simulink model "test_delfttyre_sti_cleat"  (Simulink 6.4)
settings: Solver=ode45  SolverMode=SingleTasking  StartTime=0.0  StopTime=0.5  FixedStep=0.00025  MaxStep=0.001  RelTol=1e-4  AbsTol=1e-4
values from neighbouring files (symbols this model uses):
  axle_z = typarr_struct.DIMENSION.UNLOADED_RADIUS - varinf(varinf_ptr.IDEFL)    [run_cleat_example_reduced_input_tpf.m]
  IYY_wheel = IYY-BELT_IYY+RIMROTIN+TRGROTIN    [run_cleat_example_reduced_input_tpf.m]
  Omega0 = Vx/varinf(varinf_ptr.IREF)    [run_cleat_example_reduced_input_tpf.m]
  Vx = 40/3.6    (= 11.1111111111)    [run_cleat_example_reduced_input_tpf.m]
libraries: simulink x4, Delft_Tyre_sm1glib x2, Delft_Tyre_dtlib x2
settings Model: Creator=schmeitzajc  LastModifiedBy=hofstadrhmtvd  ExtModeTrigMode=oneshot  ExtModeArmWhenConnect=off
settings SolverCC: InitialStep=0.001
settings DataIOCC: LimitDataPoints=off  SignalLoggingName=sigsOut
settings OptimizationCC: BooleanDataType=off
settings DebuggingCC: SolverPrmCheckMsg=none  StrictBusMsg=ErrorLevel1
settings HardwareCC: TargetHWDeviceType=32-bit Generic  TargetUnknown=on  ProdEqTarget=off

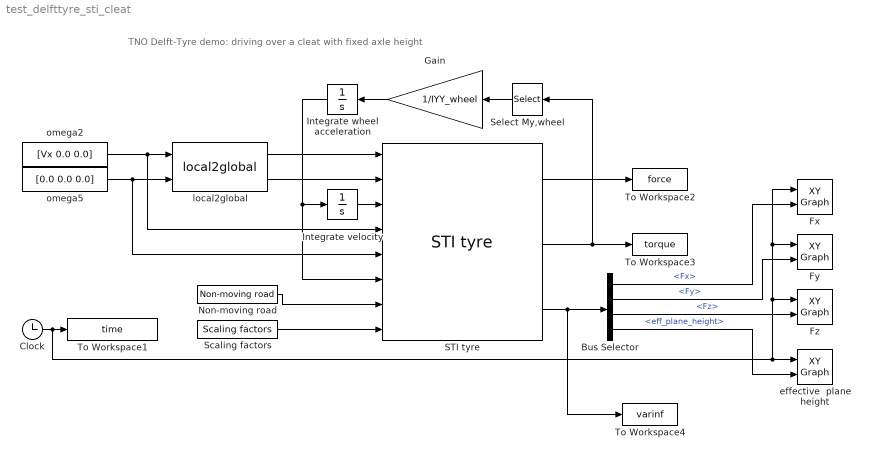
== system test_delfttyre_sti_cleat ==
  note: TNO Delft-Tyre demo: driving over a cleat with fixed axle height
  Bus Selector : BusSelector  OutputSignals=Fx,Fy,Fz,eff_plane_height
  Clock : Clock
      settings: Decimation=10
  Fx : simulink/Sinks/XY Graph  SystemSampleTime=-1  xmin=0  xmax=0.5  ymin=-2000  ymax=2000  st=-1
  Fy : simulink/Sinks/XY Graph  SystemSampleTime=-1  xmin=0  xmax=0.5  ymin=-1000  ymax=1000  st=-1
  Fz : simulink/Sinks/XY Graph  SystemSampleTime=-1  xmin=0  xmax=0.5  ymin=0  ymax=10000  st=-1
  Gain : Gain  Orientation=left  Gain=1/IYY_wheel  ParameterDataType=fixdt(1,16,0)  ParameterScaling=[]  OutDataType=fixdt(1,16,0)  OutScaling=[]
  Integrate velocity : Integrator
  Integrate wheel acceleration : Integrator  Orientation=left  InitialCondition=Omega0
  Non-moving road : Delft_Tyre_sm1glib/SimMechanics 1G/Non-moving road  Tag=Non-moving road  SystemSampleTime=-1  dummy=off
  STI tyre : Delft_Tyre_dtlib/Simulink/STI tyre  Tag=STI tyre  SystemSampleTime=-1  idtyre=1  tpfname=tpfname  rdfname=rdfname  side_mode=(3xxx) symmetric  cnt_mode=(x5xx) 3D short wavelength road contact  dyn_mode=(xx4x) rigid ring + initial statics  mf_mode=(xxx4) combined  use_mode=1e8  disp_debug=off
  Scaling factors : Delft_Tyre_sm1glib/SimMechanics 1G/Scaling factors  Tag=Scaling factors  SystemSampleTime=-1  LMUX=1  LKX=1  LMUY=1  LKY=1  LKYC=1  LTR=1  LKZC=1
  Select My,wheel : Selector  Orientation=left  Elements=2  Rows=2  InputPortWidth=3  OutputPortSize=[(-2)]
  To Workspace1 : ToWorkspace  VariableName=time  SampleTime=-1  SaveFormat=Array
  To Workspace2 : ToWorkspace  VariableName=force  SampleTime=-1  SaveFormat=Array
  To Workspace3 : ToWorkspace  VariableName=torque  SampleTime=-1  SaveFormat=Array
  To Workspace4 : ToWorkspace  VariableName=varinf  SampleTime=-1  SaveFormat=Array
  effective  plane height : simulink/Sinks/XY Graph  SystemSampleTime=-1  xmin=0  xmax=0.5  ymin=-0.05  ymax=0.05  st=-1
  local2global : Delft_Tyre_dtlib/Simulink/local2global  Tag=local2global  SystemSampleTime=-1  init_pos=[0 0 axle_z]  init_angle=[0 0 0]
  omega2 : Constant  Value=[Vx 0.0 0.0]  OutDataType=fixdt(1,16,0)  ConRadixGroup=Use specified scaling  OutScaling=[]  SampleTime=inf  FramePeriod=inf
  omega5 : Constant  Value=[0.0 0.0 0.0]  OutDataType=fixdt(1,16,0)  ConRadixGroup=Use specified scaling  OutScaling=[]  SampleTime=inf  FramePeriod=inf
  wires:
  STI tyre/1 -> To Workspace2/1
  Clock/1 -> To Workspace1/1, effective  plane height/1, Fz/1, Fx/1, Fy/1
  omega2/1 -> STI tyre/4, local2global/1
  Integrate wheel acceleration/1 -> Integrate velocity/1, STI tyre/6
  omega5/1 -> STI tyre/5, local2global/2
  STI tyre/2 -> To Workspace3/1, Select My,wheel/1
  STI tyre/3 -> Bus Selector/1, To Workspace4/1
  local2global/1 -> STI tyre/1
  local2global/2 -> STI tyre/2
  Integrate velocity/1 -> STI tyre/3
  Scaling factors/1 -> STI tyre/8
  Bus Selector/1 -> Fx/2  "<Fx>"
  Bus Selector/3 -> Fz/2  "<Fz>"
  Bus Selector/4 -> effective  plane height/2  "<eff_plane_height>"
  Bus Selector/2 -> Fy/2  "<Fy>"
  Non-moving road/1 -> STI tyre/7
  Select My,wheel/1 -> Gain/1
  Gain/1 -> Integrate wheel acceleration/1
